simulink model "single_dof"  (Simulink 8.6)
settings: Solver=VariableStepAuto  StartTime=0.0  StopTime=10  RelTol=1e-3
undefined symbols (not defined in the file or in its folder): bDevice, mDevice, p0, v0
settings Model: Creator=TOSHIBA  LastModifiedBy=TOSHIBA
settings DataIOCC: SaveFormat=Dataset  SignalLoggingSaveFormat=Dataset
settings OptimizationCC: ExpressionDepthLimit=128
settings DebuggingCC: UnderspecifiedInitializationDetection=Simplified  MergeDetectMultiDrivingBlocksExec=error  SolverPrmCheckMsg=none  FcnCallInpInsideContextMsg=EnableAllAsError  StateNameClashWarn=none
settings HardwareCC: ProdBitPerPointer=64  ProdLargestAtomicFloat=Float  ProdIntDivRoundTo=Zero  ProdEndianess=LittleEndian  ProdWordSize=64  ProdHWDeviceType=Intel->x86-64 (Windows64)
settings GRTTargetCC: GeneratePreprocessorConditionals=Use local settings  CombineOutputUpdateFcns=on  GRTInterface=off
settings ConfigComp: CovModelRefEnable=off

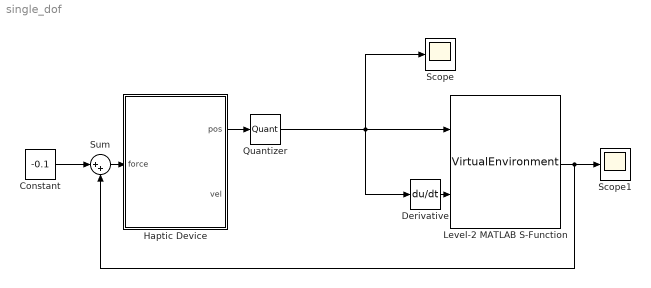
== system single_dof ==
  Constant : Constant  Value=-0.1
  Derivative : Derivative
  Haptic Device : Subsystem
  Level-2 MATLAB S-Function : M-S-Function  FunctionName=VirtualEnvironment  Parameters=kWall, bWall, nWall, pWall, dof, tsampling
  Quantizer : Quantizer  QuantizationInterval=0.00001
  Scope : Scope
  Scope1 : Scope
  Sum : Sum  Inputs=|++
  wires:
  Sum/1 -> Haptic Device/1(force)
  Level-2 MATLAB S-Function/1 -> Scope1/1, Sum/2
  Constant/1 -> Sum/1
  Derivative/1 -> Level-2 MATLAB S-Function/2
  Haptic Device/1(pos) -> Quantizer/1
  Quantizer/1 -> Scope/1, Derivative/1, Level-2 MATLAB S-Function/1

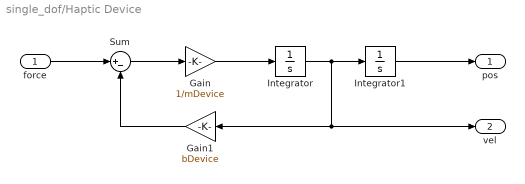
== system single_dof/Haptic Device ==
  force : Inport
  Gain : Gain  Gain=1/mDevice
  Gain1 : Gain  Gain=bDevice
  Integrator : Integrator  InitialCondition=v0
  Integrator1 : Integrator  InitialCondition=p0
  Sum : Sum  Inputs=|+-
  pos : Outport
  vel : Outport  Port=2
  wires:
  Sum/1 -> Gain/1
  Integrator/1 -> vel/1, Gain1/1, Integrator1/1
  Integrator1/1 -> pos/1
  Gain1/1 -> Sum/2
  Gain/1 -> Integrator/1
  force/1 -> Sum/1
